simulink model "pwm_bakkup"  (R2018b)
settings: Solver=FixedStepAuto  StartTime=0.0  StopTime=inf  FixedStep=.001  RelTol=1e-3  EnableMultiTasking=on
settings Model: SimulationMode=external  Creator=dskaputa  LastModifiedBy=my3197
settings SolverCC: PositivePriorityOrder=on
settings OptimizationCC: PassReuseOutputArgsAs=Individual arguments  MaxStackSize=64
settings DebuggingCC: ParameterTunabilityLossMsg=error
settings HardwareCC: ProdBitPerPointer=32  ProdBitPerSizeT=32  ProdBitPerPtrDiffT=32  ProdLargestAtomicInteger=Long  ProdLargestAtomicFloat=Double  ProdWordSize=32  ProdHWDeviceType=ARM Compatible->ARM Cortex
settings SFSimCC: SimUseLocalCustomCode=off  MATLABDynamicMemAlloc=off
settings RTWCC: SystemTargetFile=ert.tlc  HardwareBoard=Xilinx Zynq-7000 based board  TLCOptions="-aInlineSetEventsForThisBaseRateFcn=TLC_FALSE -aSuppressMultiTaskScheduler=TLC_FALSE  -aRateBasedStepFcn=0"  TemplateMakefile=ert_default_tmf  GenerateReport=on  RTWUseLocalCustomCode=off  Toolchain=Linaro AArch32 Linux v6.3.1  IncludeHyperlinkInReport=on  LaunchReport=on  GenerateTraceInfo=on  GenerateTraceReport=on  GenerateTraceReportSl=on  GenerateTraceReportSf=on  GenerateTraceReportEml=on
settings CodeAppCC: ForceParamTrailComments=on  IgnoreCustomStorageClasses=off  OperatorAnnotations=on  SimulinkDataObjDesc=on  SFDataObjDesc=on  MATLABFcnDesc=on  InsertBlockDesc=on  StateflowObjectComments=on  MATLABSourceComments=on
settings ERTTargetCC: SupportNonInlinedSFcns=on

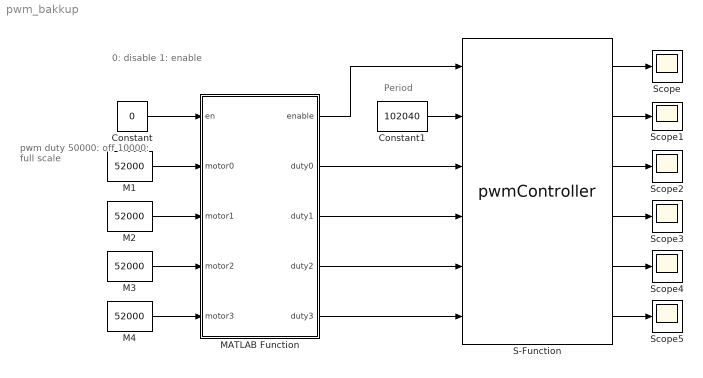
== system pwm_bakkup ==
  note: pwm duty
      | 50000: off
      | 10000: full scale
  note: 0: disable
      | 1: enable
  note: Period
  Constant : Constant  Value=0  SampleTime=-1
  Constant1 : Constant  Value=102040  SampleTime=-1
  M{1..4} (4 alike) : Constant  Value=52000  SampleTime=-1
  MATLAB Function : MATLAB Function  TreatAsAtomicUnit=on
  S-Function : S-Function  FunctionName=pwmController  SFunctionDeploymentMode=off  EnableBusSupport=off
      mask Display: image('pwm.jpg');
  Scope{,1..5} (6 alike) : Scope
  wires:
  Constant/1 -> MATLAB Function/1(en)
  S-Function/1 -> Scope/1
  S-Function/2 -> Scope1/1
  S-Function/3 -> Scope2/1
  S-Function/4 -> Scope3/1
  S-Function/5 -> Scope4/1
  Constant1/1 -> S-Function/2
  MATLAB Function/2(duty0) -> S-Function/3
  MATLAB Function/3(duty1) -> S-Function/4
  MATLAB Function/4(duty2) -> S-Function/5
  MATLAB Function/5(duty3) -> S-Function/6
  M1/1 -> MATLAB Function/2(motor0)
  M2/1 -> MATLAB Function/3(motor1)
  M3/1 -> MATLAB Function/4(motor2)
  M4/1 -> MATLAB Function/5(motor3)
  S-Function/6 -> Scope5/1
  MATLAB Function/1(enable) -> S-Function/1

== matlab function pwm_bakkup/MATLAB Function ==
  data: enable output; en input; duty0 output; duty1 output; duty2 output; duty3 output; motor0 input; motor1 input; motor2 input; motor3 input
function [enable, duty0,duty1,duty2,duty3]= fcn(en,motor0,motor1,motor2,motor3)


if (en == 0)
    duty0 = 50000;
    duty1 = 50000;
    duty2 = 50000;
    duty3 = 50000;
else
    duty0 = motor0;
    duty1 = motor1;
    duty2 = motor2;
    duty3 = motor3;
end

enable = 1;
